simulink model "mypid2"  (R2017a)
settings: Solver=VariableStepAuto  StartTime=0.0  StopTime=10.0  RelTol=1e-3
undefined symbols (not defined in the file or in its folder): s
settings Model: Creator=Grażynka  LastModifiedBy=Grażynka

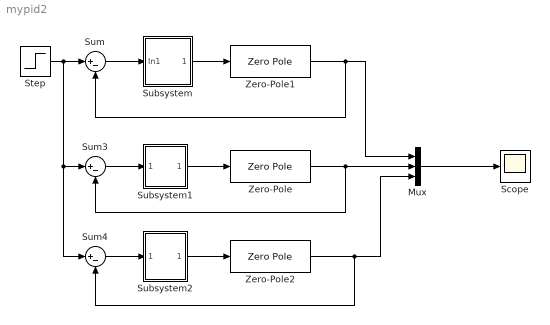
== system mypid2 ==
  Mux : Mux  Inputs=3
  Scope : Scope
  Step : Step  SampleTime=0
  Subsystem : Subsystem  mask{P=0, I=0, D=0}
  Subsystem1 : Subsystem  mask{P=0, I=0, D=0}
  Subsystem2 : Subsystem  mask{P=0, I=0, D=0}
  Sum : Sum  Inputs=|+-
  Sum3 : Sum  Inputs=|+-
  Sum4 : Sum  Inputs=|+-
  Zero-Pole : ZeroPole  Zeros=[]  Poles=[-1 -1 -1]
  Zero-Pole1 : ZeroPole  Zeros=[]  Poles=[-1 -1 -1]
  Zero-Pole2 : ZeroPole  Zeros=[]  Poles=[-1 -1 -1]
  wires:
  Step/1 -> Sum3/1, Sum4/1, Sum/1
  Subsystem/1(Out1) -> Zero-Pole1/1
  Mux/1 -> Scope/1
  Sum/1 -> Subsystem/1(In1)
  Zero-Pole1/1 -> Sum/2, Mux/1
  Sum3/1 -> Subsystem1/1(In1)
  Subsystem1/1(Out1) -> Zero-Pole/1
  Sum4/1 -> Subsystem2/1(In1)
  Subsystem2/1(Out1) -> Zero-Pole2/1
  Zero-Pole/1 -> Sum3/2, Mux/2
  Zero-Pole2/1 -> Sum4/2, Mux/3

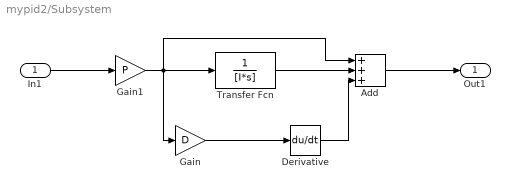
== system mypid2/Subsystem ==
  In1 : Inport
  Add : Sum  Inputs=+++
  Derivative : Derivative
  Gain : Gain  Gain=D
  Gain1 : Gain  Gain=P
  Transfer Fcn : TransferFcn  Denominator=[I*s]
  Out1 : Outport
  wires:
  Add/1 -> Out1/1
  Gain1/1 -> Gain/1, Add/1, Transfer Fcn/1
  Derivative/1 -> Add/3
  Transfer Fcn/1 -> Add/2
  In1/1 -> Gain1/1
  Gain/1 -> Derivative/1

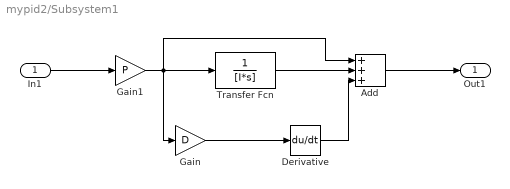
== system mypid2/Subsystem1 ==
  In1 : Inport
  Add : Sum  Inputs=+++
  Derivative : Derivative
  Gain : Gain  Gain=D
  Gain1 : Gain  Gain=P
  Transfer Fcn : TransferFcn  Denominator=[I*s]
  Out1 : Outport
  wires:
  Add/1 -> Out1/1
  Gain1/1 -> Gain/1, Add/1, Transfer Fcn/1
  Derivative/1 -> Add/3
  Transfer Fcn/1 -> Add/2
  In1/1 -> Gain1/1
  Gain/1 -> Derivative/1

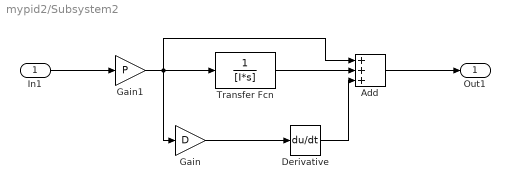
== system mypid2/Subsystem2 ==
  In1 : Inport
  Add : Sum  Inputs=+++
  Derivative : Derivative
  Gain : Gain  Gain=D
  Gain1 : Gain  Gain=P
  Transfer Fcn : TransferFcn  Denominator=[I*s]
  Out1 : Outport
  wires:
  Add/1 -> Out1/1
  Gain1/1 -> Gain/1, Add/1, Transfer Fcn/1
  Derivative/1 -> Add/3
  Transfer Fcn/1 -> Add/2
  In1/1 -> Gain1/1
  Gain/1 -> Derivative/1
